simulink model "FurutaPendulumSys_LAB"  (R2018b)
settings: Solver=VariableStepAuto  StartTime=0.0  StopTime=20  MaxStep=0.05  RelTol=1e-3
values from neighbouring files (symbols this model uses):
  A = [0 0 1 0;0 0 0 1;0 a32 0 0; 0 a42 0 0]    [main_Furuta_LAB.m]
  B = [0 0 ; 0 0; b31 b32; b41 b42 ]    [main_Furuta_LAB.m]
  C1 = [1 0 0 0]    [main_Furuta_LAB.m]
  delta_impulse = 0.1    [main_Furuta_LAB.m]
  dq0 = x0(3:4)    [main_Furuta_LAB.m]
  g = 9.81    [main_Furuta_LAB.m]
  J1 = 0.000027+0.00257    (= 0.002597)    [main_Furuta_LAB.m]
  J2 = 4.15e-5    (= 4.15e-05)    [main_Furuta_LAB.m]
  Kdrv = 2    [main_Furuta_LAB.m]
  Kinf = place(A,B(:,1),pp)    [main_Furuta_LAB.m]
  Kt = 0.071    [main_Furuta_LAB.m]
  L = place(A',C1',pp)'    [main_Furuta_LAB.m]
  l1 = 0.16    [main_Furuta_LAB.m]
  l2 = 0.15/2    (= 0.075)    [main_Furuta_LAB.m]
  m2 = 0.0206    [main_Furuta_LAB.m]
  pulse2rad = 2*pi/2000    (= 0.00314159265359)    [main_Furuta_LAB.m]
  q0 = x0(1:2)    [main_Furuta_LAB.m]
  t_impulse = 10    [main_Furuta_LAB.m]
  tau2_impulse = 0.001    [main_Furuta_LAB.m]
  Tderiv = 1/200    (= 0.005)    [main_Furuta_LAB.m]
  Vmax = 3    [main_Furuta_LAB.m]
settings Model: Creator=lucaschenato  LastModifiedBy=Luca

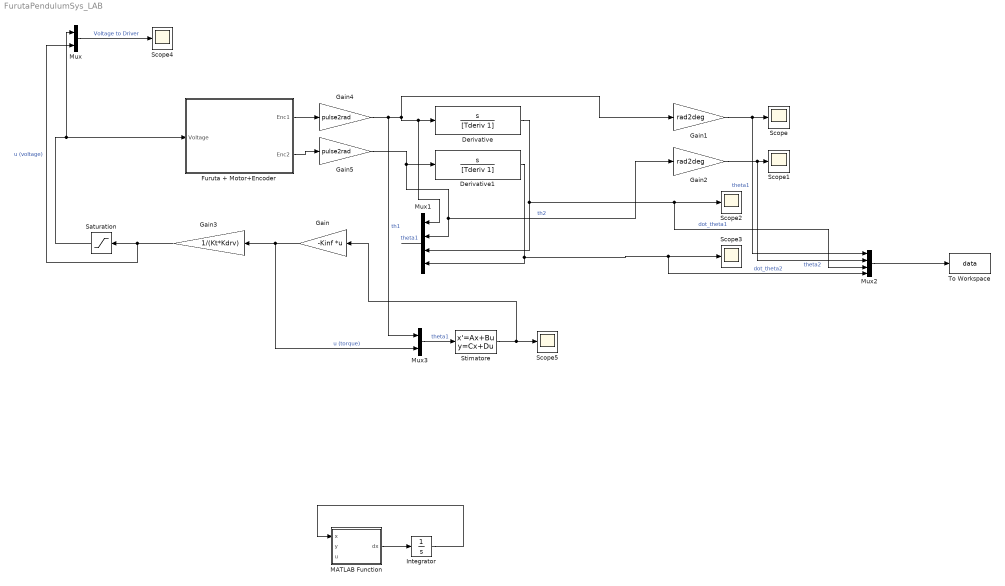
== system FurutaPendulumSys_LAB ==
  Derivative : TransferFcn  Numerator=[1 0]  Denominator=[Tderiv 1]
  Derivative1 : TransferFcn  Numerator=[1 0]  Denominator=[Tderiv 1]
  Furuta + Motor+Encoder : Subsystem
  Gain : Gain  Gain=-Kinf  Multiplication=Matrix(K*u)
  Gain1 : Gain  Gain=rad2deg
  Gain2 : Gain  Gain=rad2deg
  Gain3 : Gain  Gain=1/(Kt*Kdrv)
  Gain4 : Gain  Gain=pulse2rad
  Gain5 : Gain  Gain=pulse2rad
  Integrator : Integrator
  MATLAB Function : MATLAB Function  TreatAsAtomicUnit=on
  Mux : Mux  Inputs=2
  Mux1 : Mux
  Mux2 : Mux
  Mux3 : Mux  Inputs=2
  Saturation : Saturate  UpperLimit=Vmax  LowerLimit=-Vmax
  Scope{,1..5} (6 alike) : Scope
  Stimatore : StateSpace  A=A-L*C1  B=[L B(:,1)]  C=eye(4)  D=zeros(4,2)  InitialCondition=0
  To Workspace : ToWorkspace  VariableName=data  SaveFormat=Structure With Time  SampleTime=-1
  wires:
  Gain1/1 -> Mux2/1, Scope/1  "theta1"
  Derivative1/1 -> Mux2/4, Scope3/1, Mux1/4  "dot_theta2"
  Derivative/1 -> Mux1/3, Mux2/3, Scope2/1  "dot_theta1"
  Mux1/1 -> ?  "theta1"
  Gain4/1 -> Mux3/1, Mux1/1, Derivative/1, Gain1/1  "th1"
  Gain5/1 -> Mux1/2, Gain2/1, Derivative1/1  "th2"
  Gain2/1 -> Mux2/2, Scope1/1  "theta2"
  Gain3/1 -> Mux/2, Saturation/1  "u (voltage)"
  Gain/1 -> Mux3/2, Gain3/1  "u (torque)"
  Furuta + Motor+Encoder/1(Enc1) -> Gain4/1
  Furuta + Motor+Encoder/2(Enc2) -> Gain5/1
  Saturation/1 -> Mux/1, Furuta + Motor+Encoder/1(Voltage)
  Mux/1 -> Scope4/1  "Voltage to Driver"
  Mux2/1 -> To Workspace/1
  MATLAB Function/1(dx) -> Integrator/1
  Integrator/1 -> MATLAB Function/1(x)
  Mux3/1 -> Stimatore/1  "theta1"
  Stimatore/1 -> Scope5/1, Gain/1

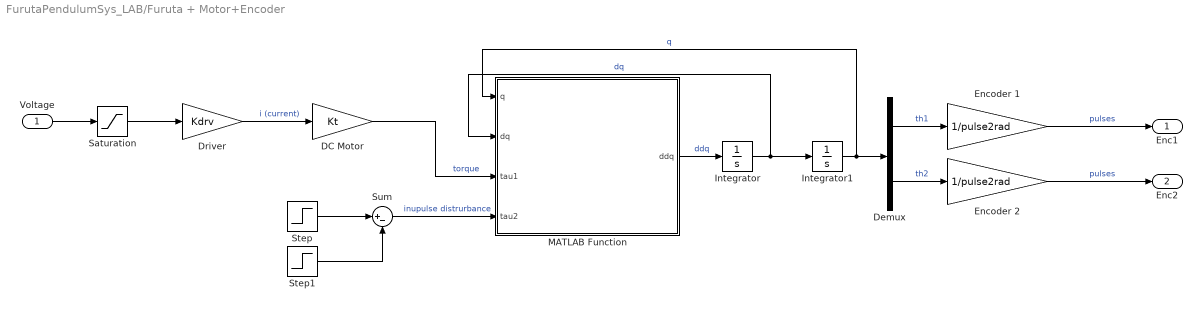
== system FurutaPendulumSys_LAB/Furuta + Motor+Encoder ==
  Voltage : Inport
  DC Motor : Gain  Gain=Kt
  Demux : Demux  Outputs=2
  Driver : Gain  Gain=Kdrv
  Encoder 1 : Gain  Gain=1/pulse2rad
  Encoder 2 : Gain  Gain=1/pulse2rad
  Integrator : Integrator  InitialCondition=dq0  ZeroCross=off
  Integrator1 : Integrator  InitialCondition=q0  ZeroCross=off
  MATLAB Function : MATLAB Function  TreatAsAtomicUnit=on
  Saturation : Saturate  UpperLimit=Vmax  LowerLimit=-Vmax
  Step : Step  Time=t_impulse  After=tau2_impulse  SampleTime=0
  Step1 : Step  Time=t_impulse+delta_impulse  After=tau2_impulse  SampleTime=0
  Sum : Sum  Inputs=|+-
  Enc1 : Outport
  Enc2 : Outport  Port=2
  wires:
  Integrator/1 -> MATLAB Function/2(dq), Integrator1/1  "dq"
  Integrator1/1 -> MATLAB Function/1(q), Demux/1  "q"
  Voltage/1 -> Saturation/1
  MATLAB Function/1(ddq) -> Integrator/1  "ddq"
  Driver/1 -> DC Motor/1  "i (current)"
  DC Motor/1 -> MATLAB Function/3(tau1)  "torque"
  Demux/1 -> Encoder 1/1  "th1"
  Demux/2 -> Encoder 2/1  "th2"
  Encoder 1/1 -> Enc1/1  "pulses"
  Encoder 2/1 -> Enc2/1  "pulses"
  Sum/1 -> MATLAB Function/4(tau2)  "inupulse distrurbance"
  Step/1 -> Sum/1
  Step1/1 -> Sum/2
  Saturation/1 -> Driver/1

== matlab function FurutaPendulumSys_LAB/MATLAB Function ==
  data: x input; y input; u input; dx output
function dx = fcn(x, y, u)

% F = [0 0 0 0; 0 0 8.7013 109.9756; 1 0 0 0; 0 1 0 0];
% G = [1;0;0;0];
% L = [29.056146939348846; 5.473045059700818e+02; 4.221298374806876e+02; 5.739828394138347e+03]
% H = [0 0 3.654883203228587e+02 5.740982543848177e+02]
% 
% dx = (F + L*H)*x - L*y + G*u;

dx = 1;

== matlab function FurutaPendulumSys_LAB/Furuta + Motor+Encoder/MATLAB Function ==
  data: q input; ddq output; dq input; tau1 input; tau2 input; J1 parameter; J2 parameter; l1 parameter; l2 parameter; m2 parameter; g parameter
function ddq = FurutaPendulum(q,dq,tau1,tau2,J1,J2,l1,l2,m2,g)

th1 = q(1); 
th2 = q(2);
dth1 = dq(1); 
dth2 = dq(2);

% Define nonlinear model: M*ddq + C*dq + G = u
M = [ J1 + m2*l1^2 + m2*l2^2*sin(th2)^2, -m2*l1*l2*cos(th2) ; ...
 -m2*l1*l2*cos(th2), J2 + m2*l2^2 ];
C = [ m2*l2^2*dth2*sin(th2)*cos(th2), ...
    m2*l2^2*dth1*sin(th2)*cos(th2) + m2*l1*l2*dth2*sin(th2); ...
     -m2*l2^2*dth1*sin(th2)*cos(th2), 0];
G = [0; -m2*l2*g*sin(th2)];

u = [tau1; tau2];

ddq = M\(-C*dq-G+u);

end
